simulink model "fullstate_servo_sim"  (R2020a)
settings: Solver=VariableStepAuto  StartTime=0.0  StopTime=30  RelTol=1e-6
undefined symbols (not defined in the file): A, B, C_full, D_full, icd, K, Ka
libraries: simulink_extras x1
settings Model: Creator=Jasper  LastModifiedBy=Jasper

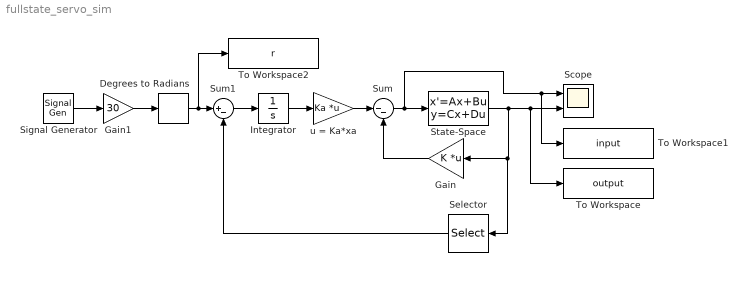
== system fullstate_servo_sim ==
  Degrees to Radians : simulink_extras/Transformations/Degrees to Radians
  Gain : Gain  Gain=K  Multiplication=Matrix(K*u)
  Gain1 : Gain  Gain=30
  Integrator : Integrator
  Scope : Scope  NumInputPorts=2
  Selector : Selector  InputPortWidth=4  IndexOptions=Index vector (dialog)  Indices=[1]  OutputSizes=1
  Signal Generator : SignalGenerator  WaveForm=square  Frequency=0.125
  State-Space : StateSpace  A=A  B=B  C=C_full  D=D_full  InitialCondition=icd
  Sum : Sum  Inputs=|--
  Sum1 : Sum  Inputs=|+-
  To Workspace : ToWorkspace  VariableName=output  SaveFormat=Timeseries  SampleTime=-1
  To Workspace1 : ToWorkspace  VariableName=input  SaveFormat=Timeseries  SampleTime=-1
  To Workspace2 : ToWorkspace  VariableName=r  SaveFormat=Timeseries  SampleTime=-1
  u = Ka*xa : Gain  Gain=Ka  Multiplication=Matrix(K*u)
  wires:
  State-Space/1 -> To Workspace/1, Scope/2, Selector/1, Gain/1
  Gain/1 -> Sum/2
  Sum/1 -> To Workspace1/1, Scope/1, State-Space/1
  Gain1/1 -> Degrees to Radians/1
  Signal Generator/1 -> Gain1/1
  Degrees to Radians/1 -> To Workspace2/1, Sum1/1
  Selector/1 -> Sum1/2
  Sum1/1 -> Integrator/1
  Integrator/1 -> u = Ka*xa/1
  u = Ka*xa/1 -> Sum/1
